simulink model "robosimulador"  (R2021b)
settings: Solver=VariableStepAuto  StartTime=0.0  StopTime=Time(length(Time))  MaxStep=1e-3  RelTol=1e-3
model workspace: external: MATLAB File /home/fabio/Desktop/Larc 2021/robosimulador_DataFile.m (data not in the file)
values from neighbouring files (symbols this model uses):
  j = length(Q)    [Cinematica_Comb.m]    (also in Cinematica_Heli_Coronal.m; Cinematica_Heli_Direta_Coronal.m; Cinematica_Heli_Sagital.m)
  Q = Qr    [Cinematica_Comb.m]
  X = zeros(1,14)    [Cinematica_Comb.m]    (also in Cinematica_Heli_Coronal.m = zeros(1,6); Cinematica_Heli_Direta_Coronal.m = zeros(1,6); Cinematica_Heli_Sagital.m = zeros(1,8))
  Y = zeros(1,14)    [Cinematica_Comb.m]    (also in Cinematica_Heli_Coronal.m = zeros(1,6); Cinematica_Heli_Direta_Coronal.m = zeros(1,6); Cinematica_Heli_Sagital.m = zeros(1,8))
  Z = zeros(1,14)    [Cinematica_Comb.m]    (also in Cinematica_Heli_Coronal.m = zeros(1,6); Cinematica_Heli_Direta_Coronal.m = zeros(1,6); Cinematica_Heli_Sagital.m = zeros(1,8))
undefined symbols (not defined in the file or in its folder): g, height_plane, plane_x, smiData, Time, Tmax, zzmp
libraries: nesl_utility x168, sm_lib x117, simulink x38, sharedutil x19, Contact_Forces_Lib x8
(part 1 of 6)
settings Model: Creator=fabio  LastModifiedBy=yurid
settings SolverCC: AlgebraicLoopSolver=TrustRegion
settings DebuggingCC: UnconnectedInputMsg=none  UnconnectedOutputMsg=none  SFMachineParentedDataDiag=warning
settings DiagnosticsConfigSet: SimMechanicsRigidlyBoundBlock=none

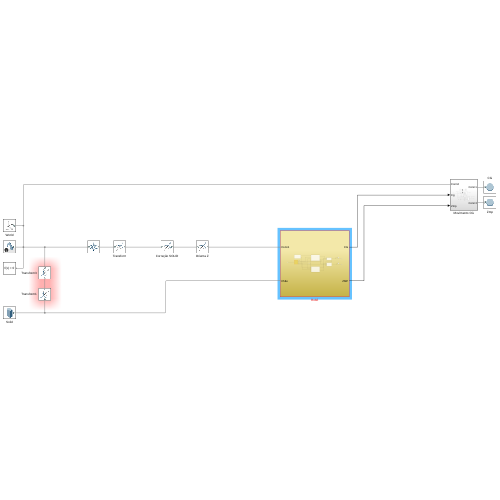
[thumbnail: Simulink's stored preview of the top-level diagram]
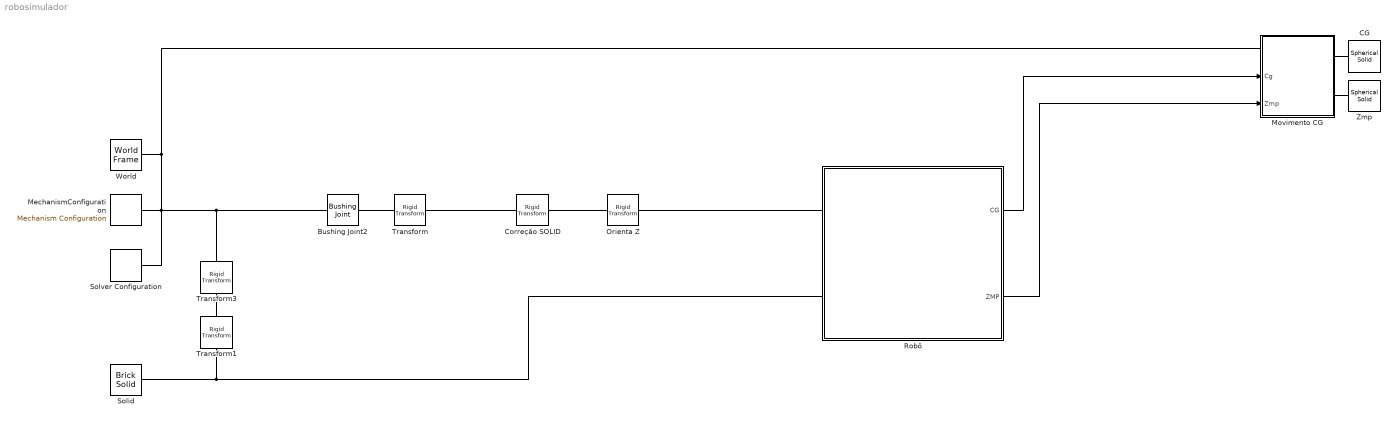
== system robosimulador ==
  Bushing Joint2 : sm_lib/Joints/Bushing Joint  JointMode=Normal  SenseConstraintForce=off  SenseConstraintForceX=off  SenseConstraintForceY=off  SenseConstraintForceZ=off  SenseConstraintTorque=off  SenseConstraintTorqueX=off  SenseConstraintTorqueY=off  SenseConstraintTorqueZ=off  SenseTotalForce=off  SenseTotalForceX=off  SenseTotalForceY=off  SenseTotalForceZ=off  SenseTotalTorque=off  SenseTotalTorqueX=off  SenseTotalTorqueY=off  SenseTotalTorqueZ=off  CompositeWrenchDir=FollowerOnBase  CompositeWrenchFrame=BaseFrame  PxEquilibriumPosition=0  PxEquilibriumPositionUnits=m  PxSpringStiffness=0  PxSpringStiffnessUnits=N/m  PxDampingCoefficient=0  PxDampingCoefficientUnits=N/(m/s)  PxTorqueActuationMode=NoTorque  PxMotionActuationMode=ComputedMotion  PxSensePosition=off  PxSenseVelocity=off  PxSenseAcceleration=off  PxSenseTorqueForce=off  PxSenseLowerLimitTorqueForce=off  PxSenseUpperLimitTorqueForce=off  PxLowerLimitSpecify=off  PxLowerLimitBound=-1  PxLowerLimitBoundUnits=m  PxLowerLimitStiffness=1e6  PxLowerLimitStiffnessUnits=N/m  PxLowerLimitDamping=1e3  PxLowerLimitDampingUnits=N/(m/s)  PxLowerLimitTransitionRegionWidth=1e-4  PxLowerLimitTransitionRegionWidthUnits=m  PxUpperLimitSpecify=off  PxUpperLimitBound=1  PxUpperLimitBoundUnits=m  PxUpperLimitStiffness=1e6  PxUpperLimitStiffnessUnits=N/m  PxUpperLimitDamping=1e3  PxUpperLimitDampingUnits=N/(m/s)  PxUpperLimitTransitionRegionWidth=1e-4  PxUpperLimitTransitionRegionWidthUnits=m  PxPositionTargetSpecify=off  PxPositionTargetPriority=High  PxPositionTargetValue=0  PxPositionTargetValueUnits=m  PxVelocityTargetSpecify=off  PxVelocityTargetPriority=High  PxVelocityTargetValue=0  PxVelocityTargetValueUnits=m/s  PyEquilibriumPosition=0  PyEquilibriumPositionUnits=m  PySpringStiffness=0  PySpringStiffnessUnits=N/m  PyDampingCoefficient=0  PyDampingCoefficientUnits=N/(m/s)  PyTorqueActuationMode=NoTorque  PyMotionActuationMode=ComputedMotion  PySensePosition=off  PySenseVelocity=off  PySenseAcceleration=off  PySenseTorqueForce=off  PySenseLowerLimitTorqueForce=off  PySenseUpperLimitTorqueForce=off  PyLowerLimitSpecify=off  PyLowerLimitBound=-1  PyLowerLimitBoundUnits=m  PyLowerLimitStiffness=1e6  PyLowerLimitStiffnessUnits=N/m  PyLowerLimitDamping=1e3  PyLowerLimitDampingUnits=N/(m/s)  PyLowerLimitTransitionRegionWidth=1e-4  PyLowerLimitTransitionRegionWidthUnits=m  PyUpperLimitSpecify=off  PyUpperLimitBound=1  PyUpperLimitBoundUnits=m  PyUpperLimitStiffness=1e6  PyUpperLimitStiffnessUnits=N/m  PyUpperLimitDamping=1e3  PyUpperLimitDampingUnits=N/(m/s)  PyUpperLimitTransitionRegionWidth=1e-4  PyUpperLimitTransitionRegionWidthUnits=m  PyPositionTargetSpecify=off  PyPositionTargetPriority=High  PyPositionTargetValue=0  PyPositionTargetValueUnits=m  PyVelocityTargetSpecify=off  PyVelocityTargetPriority=High  PyVelocityTargetValue=0  PyVelocityTargetValueUnits=m/s  PzEquilibriumPosition=0  PzEquilibriumPositionUnits=m  PzSpringStiffness=0  PzSpringStiffnessUnits=N/m  PzDampingCoefficient=0  PzDampingCoefficientUnits=N/(m/s)  PzTorqueActuationMode=NoTorque  PzMotionActuationMode=ComputedMotion  PzSensePosition=off  PzSenseVelocity=off  PzSenseAcceleration=off  PzSenseTorqueForce=off  PzSenseLowerLimitTorqueForce=off  PzSenseUpperLimitTorqueForce=off  PzLowerLimitSpecify=off  PzLowerLimitBound=-1  PzLowerLimitBoundUnits=m  PzLowerLimitStiffness=1e6  PzLowerLimitStiffnessUnits=N/m  PzLowerLimitDamping=1e3  PzLowerLimitDampingUnits=N/(m/s)  PzLowerLimitTransitionRegionWidth=1e-4  PzLowerLimitTransitionRegionWidthUnits=m  PzUpperLimitSpecify=off  PzUpperLimitBound=1  PzUpperLimitBoundUnits=m  PzUpperLimitStiffness=1e6  PzUpperLimitStiffnessUnits=N/m  PzUpperLimitDamping=1e3  PzUpperLimitDampingUnits=N/(m/s)  PzUpperLimitTransitionRegionWidth=1e-4  PzUpperLimitTransitionRegionWidthUnits=m  PzPositionTargetSpecify=off  PzPositionTargetPriority=High  PzPositionTargetValue=1  PzPositionTargetValueUnits=m  PzVelocityTargetSpecify=off  PzVelocityTargetPriority=High  PzVelocityTargetValue=0  PzVelocityTargetValueUnits=m/s  RxEquilibriumPosition=0  RxEquilibriumPositionUnits=deg  RxSpringStiffness=0  RxSpringStiffnessUnits=N*m/deg  RxDampingCoefficient=0  RxDampingCoefficientUnits=N*m/(deg/s)  RxTorqueActuationMode=NoTorque  RxMotionActuationMode=ComputedMotion  RxSensePosition=off  RxSenseVelocity=off  RxSenseAcceleration=off  RxSenseTorqueForce=off  RxSenseLowerLimitTorqueForce=off  RxSenseUpperLimitTorqueForce=off  RxLowerLimitSpecify=off  RxLowerLimitBound=-90  RxLowerLimitBoundUnits=deg  RxLowerLimitStiffness=1e4  RxLowerLimitStiffnessUnits=N*m/deg  RxLowerLimitDamping=10  RxLowerLimitDampingUnits=N*m/(deg/s)  RxLowerLimitTransitionRegionWidth=0.1  RxLowerLimitTransitionRegionWidthUnits=deg  RxUpperLimitSpecify=off  RxUpperLimitBound=90  RxUpperLimitBoundUnits=deg  RxUpperLimitStiffness=1e4  RxUpperLimitStiffnessUnits=N*m/deg  RxUpperLimitDamping=10  RxUpperLimitDampingUnits=N*m/(deg/s)  RxUpperLimitTransitionRegionWidth=0.1  RxUpperLimitTransitionRegionWidthUnits=deg  RxPositionTargetSpecify=off  RxPositionTargetPriority=High  RxPositionTargetValue=0  RxPositionTargetValueUnits=deg  RxVelocityTargetSpecify=off  RxVelocityTargetPriority=High  RxVelocityTargetValue=0  RxVelocityTargetValueUnits=deg/s  RyEquilibriumPosition=0  RyEquilibriumPositionUnits=deg  RySpringStiffness=0  RySpringStiffnessUnits=N*m/deg  RyDampingCoefficient=0  RyDampingCoefficientUnits=N*m/(deg/s)  RyTorqueActuationMode=NoTorque  RyMotionActuationMode=ComputedMotion  RySensePosition=off  RySenseVelocity=off  RySenseAcceleration=off  RySenseTorqueForce=off  RySenseLowerLimitTorqueForce=off  RySenseUpperLimitTorqueForce=off  RyLowerLimitSpecify=off  RyLowerLimitBound=-90  RyLowerLimitBoundUnits=deg  RyLowerLimitStiffness=1e4  RyLowerLimitStiffnessUnits=N*m/deg  RyLowerLimitDamping=10  RyLowerLimitDampingUnits=N*m/(deg/s)  RyLowerLimitTransitionRegionWidth=0.1  RyLowerLimitTransitionRegionWidthUnits=deg  RyUpperLimitSpecify=off  RyUpperLimitBound=90  RyUpperLimitBoundUnits=deg  RyUpperLimitStiffness=1e4  RyUpperLimitStiffnessUnits=N*m/deg  RyUpperLimitDamping=10  RyUpperLimitDampingUnits=N*m/(deg/s)  RyUpperLimitTransitionRegionWidth=0.1  RyUpperLimitTransitionRegionWidthUnits=deg  RyPositionTargetSpecify=off  RyPositionTargetPriority=High  RyPositionTargetValue=0  RyPositionTargetValueUnits=deg  RyVelocityTargetSpecify=off  RyVelocityTargetPriority=High  RyVelocityTargetValue=0  RyVelocityTargetValueUnits=deg/s  RzEquilibriumPosition=0  RzEquilibriumPositionUnits=deg  RzSpringStiffness=0  RzSpringStiffnessUnits=N*m/deg  RzDampingCoefficient=0  RzDampingCoefficientUnits=N*m/(deg/s)  RzTorqueActuationMode=NoTorque  RzMotionActuationMode=ComputedMotion  RzSensePosition=off  RzSenseVelocity=off  RzSenseAcceleration=off  RzSenseTorqueForce=off  RzSenseLowerLimitTorqueForce=off  RzSenseUpperLimitTorqueForce=off  RzLowerLimitSpecify=off  RzLowerLimitBound=-90  RzLowerLimitBoundUnits=deg  RzLowerLimitStiffness=1e4  RzLowerLimitStiffnessUnits=N*m/deg  RzLowerLimitDamping=10  RzLowerLimitDampingUnits=N*m/(deg/s)  RzLowerLimitTransitionRegionWidth=0.1  RzLowerLimitTransitionRegionWidthUnits=deg  RzUpperLimitSpecify=off  RzUpperLimitBound=90  RzUpperLimitBoundUnits=deg  RzUpperLimitStiffness=1e4  RzUpperLimitStiffnessUnits=N*m/deg  RzUpperLimitDamping=10  RzUpperLimitDampingUnits=N*m/(deg/s)  RzUpperLimitTransitionRegionWidth=0.1  RzUpperLimitTransitionRegionWidthUnits=deg  RzPositionTargetSpecify=off  RzPositionTargetPriority=High  RzPositionTargetValue=0  RzPositionTargetValueUnits=deg  RzVelocityTargetSpecify=off  RzVelocityTargetPriority=High  RzVelocityTargetValue=0  RzVelocityTargetValueUnits=deg/s
  CG : sm_lib/Body Elements/Spherical Solid  GraphicAmbientColor=[0.15 0.15 0.15 1.0]  BasedOnType=Density  CenterOfMass=[0 0 0]  CenterOfMassUnits=m  GraphicDiffuseColor=[0.2 1.0 0.0]  Density=1000  DensityUnits=kg/m^3  DoExposeReferenceFrame=on  GraphicEmissiveColor=[0.0 0.0 0.0 1.0]  ExportEntireGeometry=off  SerializedExposedGeometries=<ExposedGeometries/>  SerializedFrames=<Frames/>  MarkerShape=Sphere  MarkerSize=10  GraphicType=FromGeometry  InertiaType=CalculateFromGeometry  Mass=1  MassUnits=kg  MomentsOfInertia=[1 1 1]  MomentsOfInertiaUnits=kg*m^2  GraphicOpacity=1.0  ProductsOfInertia=[0 0 0]  ProductsOfInertiaUnits=kg*m^2  GraphicShininess=75  GraphicSpecularColor=[0.5 0.5 0.5 1.0]  SphereRadius=0.01  SphereRadiusUnits=m  GraphicVisPropType=SimpleVisualProperties
  Correção SOLID : sm_lib/Frames and Transforms/Rigid Transform  TranslationMethod=None  TranslationStandardOffset=0  TranslationLengthUnit=mm  TranslationStandardAxis=+Z  TranslationCartesianOffset=0  TranslationROffset=0  TranslationROffsetUnits=m  TranslationZOffset=0  TranslationZOffsetUnits=m  TranslationThetaOffset=0  TranslationThetaOffsetUnits=deg  RotationMethod=StandardAxis  RotationAngleUnits=deg  RotationStandardAxis=-Z  RotationAngle=13.6  RotationArbitraryAxis=0  FollAlignAxisA=+X  BaseAlignAxisA=+Y  FollAlignAxisB=+Y  BaseAlignAxisB=+Z  RotationSequenceAxes=FollowerAxes  RotationSequence=XYX  RotationSequenceAngles=[0 0 0]  RotationSequenceAnglesUnits=deg  RotationMatrix=[1 0 0; 0 1 0; 0 0 1]
  MechanismConfiguration : sm_lib/Utilities/Mechanism Configuration  UniformGravity=Constant  GravityVector=[0 0 -9.80665]  GravityUnits=m/s^2  LinearizationDelta=0.001  JointModeTransitionNonlinearIterations=2
  Movimento CG : Subsystem
      settings: PortSchema="{\"entries\":[{\"content\":{\"sides\":[{\"content\":{\"connectorIds\":[\"LConn1\",\"In1\",\"In2\"]},\"type\":\"ConnectorPlacement.EquallySpacedRectSide\",\"uuid\":\"e9e729ac-da44-45ac-96b7-74b9933617c8\"},{\"content\":{\"connectorIds\":[\"RConn1\",\"RConn2\"],\"side\":\"RIGHT\"},\"type\":\"ConnectorPlacement.EquallySpacedRectSide\",\"uuid\":\"b7965d14-34ef-45b5-990a-29849adbef07\"},{\"content\":{\"connectorIds\":[],\"side\":\"TOP\"},\"type\":\"ConnectorPlacement.EquallySpacedRectSide\",\"uuid\":\"174ef9aa-3bee-4810-8e13-2d3bbeb9af5d\"}]},\"type\":\"ConnectorPlacement.EquallySpacedConnector\",\"uuid\":\"22440da4-e6bb-4652-99bb-446a9d9c0133\"}],\"packageUris\":[\"http://schema.mathworks.com/mf0/Connector/R2020b\"],\"version\":\"1.0\"}"
  Orienta Z : sm_lib/Frames and Transforms/Rigid Transform  TranslationMethod=None  TranslationStandardOffset=0  TranslationLengthUnit=mm  TranslationStandardAxis=+Z  TranslationCartesianOffset=0  TranslationROffset=0  TranslationROffsetUnits=m  TranslationZOffset=0  TranslationZOffsetUnits=m  TranslationThetaOffset=0  TranslationThetaOffsetUnits=deg  RotationMethod=StandardAxis  RotationAngleUnits=deg  RotationStandardAxis=+Z  RotationAngle=90  RotationArbitraryAxis=0  FollAlignAxisA=+X  BaseAlignAxisA=+Y  FollAlignAxisB=+Y  BaseAlignAxisB=+Z  RotationSequenceAxes=FollowerAxes  RotationSequence=XYX  RotationSequenceAngles=[0 0 0]  RotationSequenceAnglesUnits=deg  RotationMatrix=[1 0 0; 0 1 0; 0 0 1]
  Robô : Subsystem
  Solid : sm_lib/Body Elements/Brick Solid  GraphicAmbientColor=[0.15 0.15 0.15 1.0]  BasedOnType=Density  BrickDimensions=chao  BrickDimensionUnits=m  CenterOfMass=[0 0 0]  CenterOfMassUnits=m  GraphicDiffuseColor=[0.5 0.5 0.5]  Density=1000  DensityUnits=kg/m^3  DoExposeReferenceFrame=on  GraphicEmissiveColor=[0.0 0.0 0.0 1.0]  ExportEntireGeometry=off  SerializedFrames=<Frames/>  MarkerShape=Sphere  MarkerSize=10  GraphicType=FromGeometry  InertiaType=CalculateFromGeometry  Mass=1  MassUnits=kg  MomentsOfInertia=[1 1 1]  MomentsOfInertiaUnits=kg*m^2  GraphicOpacity=1.0  ProductsOfInertia=[0 0 0]  ProductsOfInertiaUnits=kg*m^2  GraphicShininess=75  GraphicSpecularColor=[0.5 0.5 0.5 1.0]  GraphicVisPropType=SimpleVisualProperties
  Solver Configuration : nesl_utility/Solver Configuration  PhysicalDomain=network_engine_domain  SubClassName=solver  LeftPortType=input  RightPortType=generic  Tones=[]  Harmonics=[]  SimulateNoise=off  Profile=off  UseLocalSampling=off  EnableSwitchedLinearOptims=on  FrequencyDomain=off  UseCCode=off  RelTol=0.001  AbsTol=1e-06  MinStep=1e-09  ToWorkspace=off  RevertToSquareIcSolve=off  NumHomotopyIterations=100  PhasorMode=off  PhasorModeNumHarmonics=1  DoDC=off  ResidualTolerance=1e-09  UseLocalSolver=off  LocalSolverChoice=NE_BACKWARD_EULER_ADVANCER  LocalSolverSampleTime=0.001  DoFixedCost=off  MaxNonlinIter=3  MaxModeIter=2  ComputeImpulses=off  ImpulseIterations=2  LinearAlgebra=auto  EquationFormulation=NE_TIME_EF  DelaysMemoryBudget=1024  AutomaticFiltering=on  FilteringTimeConstant=0.001  PartitionStorageMethod=AS_NEEDED  PartitionMemoryBudget=1024  PartitionMethod=ROBUST
      settings: SourceProductBaseCode=PW,SS
  Transform : sm_lib/Frames and Transforms/Rigid Transform  TranslationMethod=Cartesian  TranslationStandardOffset=0  TranslationLengthUnit=mm  TranslationStandardAxis=+Z  TranslationCartesianOffset=smiData.RigidTransform(37).translation  TranslationROffset=0  TranslationROffsetUnits=m  TranslationZOffset=0  TranslationZOffsetUnits=m  TranslationThetaOffset=0  TranslationThetaOffsetUnits=deg  RotationMethod=ArbitraryAxis  RotationAngleUnits=rad  RotationStandardAxis=+Z  RotationAngle=smiData.RigidTransform(37).angle  RotationArbitraryAxis=smiData.RigidTransform(37).axis  FollAlignAxisA=+X  BaseAlignAxisA=+Y  FollAlignAxisB=+Y  BaseAlignAxisB=+Z  RotationSequenceAxes=FollowerAxes  RotationSequence=XYX  RotationSequenceAngles=[0 0 0]  RotationSequenceAnglesUnits=deg  RotationMatrix=[1 0 0; 0 1 0; 0 0 1]
  Transform1 : sm_lib/Frames and Transforms/Rigid Transform  TranslationMethod=StandardAxis  TranslationStandardOffset=plane_x/2-0.2  TranslationLengthUnit=m  TranslationStandardAxis=+X  TranslationCartesianOffset=0.2  TranslationROffset=0  TranslationROffsetUnits=m  TranslationZOffset=0  TranslationZOffsetUnits=m  TranslationThetaOffset=0  TranslationThetaOffsetUnits=deg  RotationMethod=None  RotationAngleUnits=deg  RotationStandardAxis=+X  RotationAngle=90  RotationArbitraryAxis=smiData.RigidTransform(23).axis  FollAlignAxisA=+X  BaseAlignAxisA=+Y  FollAlignAxisB=+Y  BaseAlignAxisB=+Z  RotationSequenceAxes=FollowerAxes  RotationSequence=XYX  RotationSequenceAngles=[0 0 0]  RotationSequenceAnglesUnits=deg  RotationMatrix=[1 0 0; 0 1 0; 0 0 1]
  Transform3 : sm_lib/Frames and Transforms/Rigid Transform  TranslationMethod=StandardAxis  TranslationStandardOffset=dz  TranslationLengthUnit=m  TranslationStandardAxis=+Z  TranslationCartesianOffset=0.2  TranslationROffset=0  TranslationROffsetUnits=m  TranslationZOffset=0  TranslationZOffsetUnits=m  TranslationThetaOffset=0  TranslationThetaOffsetUnits=deg  RotationMethod=None  RotationAngleUnits=deg  RotationStandardAxis=+X  RotationAngle=90  RotationArbitraryAxis=smiData.RigidTransform(23).axis  FollAlignAxisA=+X  BaseAlignAxisA=+Y  FollAlignAxisB=+Y  BaseAlignAxisB=+Z  RotationSequenceAxes=FollowerAxes  RotationSequence=XYX  RotationSequenceAngles=[0 0 0]  RotationSequenceAnglesUnits=deg  RotationMatrix=[1 0 0; 0 1 0; 0 0 1]
  World : sm_lib/Frames and Transforms/World Frame
  Zmp : sm_lib/Body Elements/Spherical Solid  GraphicAmbientColor=[0.15 0.15 0.15 1.0]  BasedOnType=Density  CenterOfMass=[0 0 0]  CenterOfMassUnits=m  GraphicDiffuseColor=[1.0 0.0 0.0]  Density=1000  DensityUnits=kg/m^3  DoExposeReferenceFrame=on  GraphicEmissiveColor=[0.0 0.0 0.0 1.0]  ExportEntireGeometry=off  SerializedExposedGeometries=<ExposedGeometries/>  SerializedFrames=<Frames/>  MarkerShape=Sphere  MarkerSize=10  GraphicType=FromGeometry  InertiaType=CalculateFromGeometry  Mass=1  MassUnits=kg  MomentsOfInertia=[1 1 1]  MomentsOfInertiaUnits=kg*m^2  GraphicOpacity=1.0  ProductsOfInertia=[0 0 0]  ProductsOfInertiaUnits=kg*m^2  GraphicShininess=75  GraphicSpecularColor=[0.5 0.5 0.5 1.0]  SphereRadius=0.01  SphereRadiusUnits=m  GraphicVisPropType=SimpleVisualProperties
  wires:
  Robô/2(ZMP) -> Movimento CG/2(Zmp)
  Robô/1(CG) -> Movimento CG/1(Cg)
  connections:
  MechanismConfiguration/RConn1 -- Solver Configuration/RConn1 -- Movimento CG/LConn1 -- World/RConn1 -- Bushing Joint2/LConn1 -- Transform3/LConn1
  Robô/LConn1 -- Orienta Z/RConn1
  Correção SOLID/LConn1 -- Transform/RConn1
  Orienta Z/LConn1 -- Correção SOLID/RConn1
  Transform3/RConn1 -- Transform1/LConn1
  Transform1/RConn1 -- Robô/LConn2 -- Solid/RConn1
  Bushing Joint2/RConn1 -- Transform/LConn1
  CG/RConn1 -- Movimento CG/RConn1
  Zmp/RConn1 -- Movimento CG/RConn2

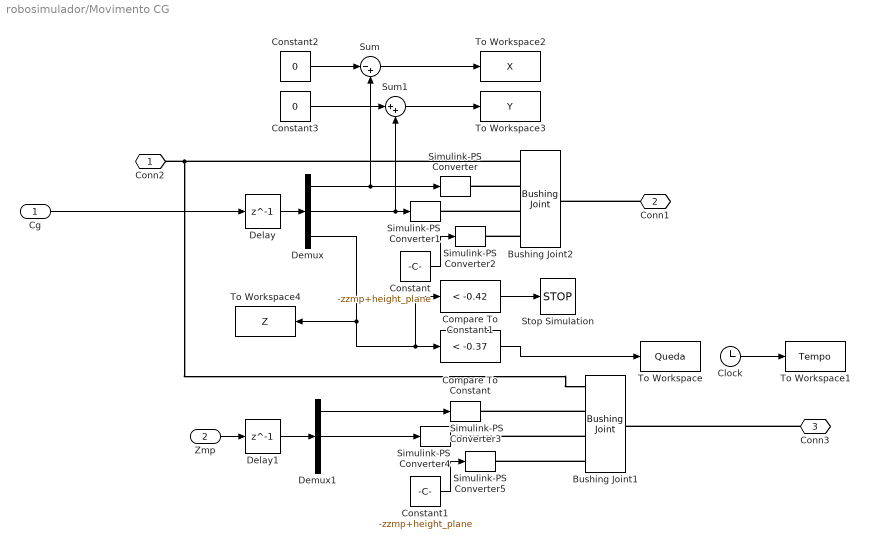
== system robosimulador/Movimento CG ==
  Cg : Inport
  Zmp : Inport  Port=2
  Bushing Joint1 : sm_lib/Joints/Bushing Joint  JointMode=Normal  SenseConstraintForce=off  SenseConstraintForceX=off  SenseConstraintForceY=off  SenseConstraintForceZ=off  SenseConstraintTorque=off  SenseConstraintTorqueX=off  SenseConstraintTorqueY=off  SenseConstraintTorqueZ=off  SenseTotalForce=off  SenseTotalForceX=off  SenseTotalForceY=off  SenseTotalForceZ=off  SenseTotalTorque=off  SenseTotalTorqueX=off  SenseTotalTorqueY=off  SenseTotalTorqueZ=off  CompositeWrenchDir=FollowerOnBase  CompositeWrenchFrame=BaseFrame  PxEquilibriumPosition=0  PxEquilibriumPositionUnits=m  PxSpringStiffness=0  PxSpringStiffnessUnits=N/m  PxDampingCoefficient=0  PxDampingCoefficientUnits=N/(m/s)  PxTorqueActuationMode=ComputedTorque  PxMotionActuationMode=InputMotion  PxSensePosition=off  PxSenseVelocity=off  PxSenseAcceleration=off  PxSenseTorqueForce=off  PxSenseLowerLimitTorqueForce=off  PxSenseUpperLimitTorqueForce=off  PxLowerLimitSpecify=off  PxLowerLimitBound=-1  PxLowerLimitBoundUnits=m  PxLowerLimitStiffness=1e6  PxLowerLimitStiffnessUnits=N/m  PxLowerLimitDamping=1e3  PxLowerLimitDampingUnits=N/(m/s)  PxLowerLimitTransitionRegionWidth=1e-4  PxLowerLimitTransitionRegionWidthUnits=m  PxUpperLimitSpecify=off  PxUpperLimitBound=1  PxUpperLimitBoundUnits=m  PxUpperLimitStiffness=1e6  PxUpperLimitStiffnessUnits=N/m  PxUpperLimitDamping=1e3  PxUpperLimitDampingUnits=N/(m/s)  PxUpperLimitTransitionRegionWidth=1e-4  PxUpperLimitTransitionRegionWidthUnits=m  PxPositionTargetSpecify=off  PxPositionTargetPriority=High  PxPositionTargetValue=0  PxPositionTargetValueUnits=m  PxVelocityTargetSpecify=off  PxVelocityTargetPriority=High  PxVelocityTargetValue=0  PxVelocityTargetValueUnits=m/s  PyEquilibriumPosition=0  PyEquilibriumPositionUnits=m  PySpringStiffness=0  PySpringStiffnessUnits=N/m  PyDampingCoefficient=0  PyDampingCoefficientUnits=N/(m/s)  PyTorqueActuationMode=ComputedTorque  PyMotionActuationMode=InputMotion  PySensePosition=off  PySenseVelocity=off  PySenseAcceleration=off  PySenseTorqueForce=off  PySenseLowerLimitTorqueForce=off  PySenseUpperLimitTorqueForce=off  PyLowerLimitSpecify=off  PyLowerLimitBound=-1  PyLowerLimitBoundUnits=m  PyLowerLimitStiffness=1e6  PyLowerLimitStiffnessUnits=N/m  PyLowerLimitDamping=1e3  PyLowerLimitDampingUnits=N/(m/s)  PyLowerLimitTransitionRegionWidth=1e-4  PyLowerLimitTransitionRegionWidthUnits=m  PyUpperLimitSpecify=off  PyUpperLimitBound=1  PyUpperLimitBoundUnits=m  PyUpperLimitStiffness=1e6  PyUpperLimitStiffnessUnits=N/m  PyUpperLimitDamping=1e3  PyUpperLimitDampingUnits=N/(m/s)  PyUpperLimitTransitionRegionWidth=1e-4  PyUpperLimitTransitionRegionWidthUnits=m  PyPositionTargetSpecify=off  PyPositionTargetPriority=High  PyPositionTargetValue=0  PyPositionTargetValueUnits=m  PyVelocityTargetSpecify=off  PyVelocityTargetPriority=High  PyVelocityTargetValue=0  PyVelocityTargetValueUnits=m/s  PzEquilibriumPosition=0  PzEquilibriumPositionUnits=m  PzSpringStiffness=0  PzSpringStiffnessUnits=N/m  PzDampingCoefficient=0  PzDampingCoefficientUnits=N/(m/s)  PzTorqueActuationMode=ComputedTorque  PzMotionActuationMode=InputMotion  PzSensePosition=off  PzSenseVelocity=off  PzSenseAcceleration=off  PzSenseTorqueForce=off  PzSenseLowerLimitTorqueForce=off  PzSenseUpperLimitTorqueForce=off  PzLowerLimitSpecify=off  PzLowerLimitBound=-1  PzLowerLimitBoundUnits=m  PzLowerLimitStiffness=1e6  PzLowerLimitStiffnessUnits=N/m  PzLowerLimitDamping=1e3  PzLowerLimitDampingUnits=N/(m/s)  PzLowerLimitTransitionRegionWidth=1e-4  PzLowerLimitTransitionRegionWidthUnits=m  PzUpperLimitSpecify=off  PzUpperLimitBound=1  PzUpperLimitBoundUnits=m  PzUpperLimitStiffness=1e6  PzUpperLimitStiffnessUnits=N/m  PzUpperLimitDamping=1e3  PzUpperLimitDampingUnits=N/(m/s)  PzUpperLimitTransitionRegionWidth=1e-4  PzUpperLimitTransitionRegionWidthUnits=m  PzPositionTargetSpecify=off  PzPositionTargetPriority=High  PzPositionTargetValue=1  PzPositionTargetValueUnits=m  PzVelocityTargetSpecify=off  PzVelocityTargetPriority=High  PzVelocityTargetValue=0  PzVelocityTargetValueUnits=m/s  RxEquilibriumPosition=0  RxEquilibriumPositionUnits=deg  RxSpringStiffness=0  RxSpringStiffnessUnits=N*m/deg  RxDampingCoefficient=0  RxDampingCoefficientUnits=N*m/(deg/s)  RxTorqueActuationMode=NoTorque  RxMotionActuationMode=ComputedMotion  RxSensePosition=off  RxSenseVelocity=off  RxSenseAcceleration=off  RxSenseTorqueForce=off  RxSenseLowerLimitTorqueForce=off  RxSenseUpperLimitTorqueForce=off  RxLowerLimitSpecify=off  RxLowerLimitBound=-90  RxLowerLimitBoundUnits=deg  RxLowerLimitStiffness=1e4  RxLowerLimitStiffnessUnits=N*m/deg  RxLowerLimitDamping=10  RxLowerLimitDampingUnits=N*m/(deg/s)  RxLowerLimitTransitionRegionWidth=0.1  RxLowerLimitTransitionRegionWidthUnits=deg  RxUpperLimitSpecify=off  RxUpperLimitBound=90  RxUpperLimitBoundUnits=deg  RxUpperLimitStiffness=1e4  RxUpperLimitStiffnessUnits=N*m/deg  RxUpperLimitDamping=10  RxUpperLimitDampingUnits=N*m/(deg/s)  RxUpperLimitTransitionRegionWidth=0.1  RxUpperLimitTransitionRegionWidthUnits=deg  RxPositionTargetSpecify=off  RxPositionTargetPriority=High  RxPositionTargetValue=0  RxPositionTargetValueUnits=deg  RxVelocityTargetSpecify=off  RxVelocityTargetPriority=High  RxVelocityTargetValue=0  RxVelocityTargetValueUnits=deg/s  RyEquilibriumPosition=0  RyEquilibriumPositionUnits=deg  RySpringStiffness=0  RySpringStiffnessUnits=N*m/deg  RyDampingCoefficient=0  RyDampingCoefficientUnits=N*m/(deg/s)  RyTorqueActuationMode=NoTorque  RyMotionActuationMode=ComputedMotion  RySensePosition=off  RySenseVelocity=off  RySenseAcceleration=off  RySenseTorqueForce=off  RySenseLowerLimitTorqueForce=off  RySenseUpperLimitTorqueForce=off  RyLowerLimitSpecify=off  RyLowerLimitBound=-90  RyLowerLimitBoundUnits=deg  RyLowerLimitStiffness=1e4  RyLowerLimitStiffnessUnits=N*m/deg  RyLowerLimitDamping=10  RyLowerLimitDampingUnits=N*m/(deg/s)  RyLowerLimitTransitionRegionWidth=0.1  RyLowerLimitTransitionRegionWidthUnits=deg  RyUpperLimitSpecify=off  RyUpperLimitBound=90  RyUpperLimitBoundUnits=deg  RyUpperLimitStiffness=1e4  RyUpperLimitStiffnessUnits=N*m/deg  RyUpperLimitDamping=10  RyUpperLimitDampingUnits=N*m/(deg/s)  RyUpperLimitTransitionRegionWidth=0.1  RyUpperLimitTransitionRegionWidthUnits=deg  RyPositionTargetSpecify=off  RyPositionTargetPriority=High  RyPositionTargetValue=0  RyPositionTargetValueUnits=deg  RyVelocityTargetSpecify=off  RyVelocityTargetPriority=High  RyVelocityTargetValue=0  RyVelocityTargetValueUnits=deg/s  RzEquilibriumPosition=0  RzEquilibriumPositionUnits=deg  RzSpringStiffness=0  RzSpringStiffnessUnits=N*m/deg  RzDampingCoefficient=0  RzDampingCoefficientUnits=N*m/(deg/s)  RzTorqueActuationMode=NoTorque  RzMotionActuationMode=ComputedMotion  RzSensePosition=off  RzSenseVelocity=off  RzSenseAcceleration=off  RzSenseTorqueForce=off  RzSenseLowerLimitTorqueForce=off  RzSenseUpperLimitTorqueForce=off  RzLowerLimitSpecify=off  RzLowerLimitBound=-90  RzLowerLimitBoundUnits=deg  RzLowerLimitStiffness=1e4  RzLowerLimitStiffnessUnits=N*m/deg  RzLowerLimitDamping=10  RzLowerLimitDampingUnits=N*m/(deg/s)  RzLowerLimitTransitionRegionWidth=0.1  RzLowerLimitTransitionRegionWidthUnits=deg  RzUpperLimitSpecify=off  RzUpperLimitBound=90  RzUpperLimitBoundUnits=deg  RzUpperLimitStiffness=1e4  RzUpperLimitStiffnessUnits=N*m/deg  RzUpperLimitDamping=10  RzUpperLimitDampingUnits=N*m/(deg/s)  RzUpperLimitTransitionRegionWidth=0.1  RzUpperLimitTransitionRegionWidthUnits=deg  RzPositionTargetSpecify=off  RzPositionTargetPriority=High  RzPositionTargetValue=0  RzPositionTargetValueUnits=deg  RzVelocityTargetSpecify=off  RzVelocityTargetPriority=High  RzVelocityTargetValue=0  RzVelocityTargetValueUnits=deg/s
  Bushing Joint2 : sm_lib/Joints/Bushing Joint  JointMode=Normal  SenseConstraintForce=off  SenseConstraintForceX=off  SenseConstraintForceY=off  SenseConstraintForceZ=off  SenseConstraintTorque=off  SenseConstraintTorqueX=off  SenseConstraintTorqueY=off  SenseConstraintTorqueZ=off  SenseTotalForce=off  SenseTotalForceX=off  SenseTotalForceY=off  SenseTotalForceZ=off  SenseTotalTorque=off  SenseTotalTorqueX=off  SenseTotalTorqueY=off  SenseTotalTorqueZ=off  CompositeWrenchDir=FollowerOnBase  CompositeWrenchFrame=BaseFrame  PxEquilibriumPosition=0  PxEquilibriumPositionUnits=m  PxSpringStiffness=0  PxSpringStiffnessUnits=N/m  PxDampingCoefficient=0  PxDampingCoefficientUnits=N/(m/s)  PxTorqueActuationMode=ComputedTorque  PxMotionActuationMode=InputMotion  PxSensePosition=off  PxSenseVelocity=off  PxSenseAcceleration=off  PxSenseTorqueForce=off  PxSenseLowerLimitTorqueForce=off  PxSenseUpperLimitTorqueForce=off  PxLowerLimitSpecify=off  PxLowerLimitBound=-1  PxLowerLimitBoundUnits=m  PxLowerLimitStiffness=1e6  PxLowerLimitStiffnessUnits=N/m  PxLowerLimitDamping=1e3  PxLowerLimitDampingUnits=N/(m/s)  PxLowerLimitTransitionRegionWidth=1e-4  PxLowerLimitTransitionRegionWidthUnits=m  PxUpperLimitSpecify=off  PxUpperLimitBound=1  PxUpperLimitBoundUnits=m  PxUpperLimitStiffness=1e6  PxUpperLimitStiffnessUnits=N/m  PxUpperLimitDamping=1e3  PxUpperLimitDampingUnits=N/(m/s)  PxUpperLimitTransitionRegionWidth=1e-4  PxUpperLimitTransitionRegionWidthUnits=m  PxPositionTargetSpecify=off  PxPositionTargetPriority=High  PxPositionTargetValue=0  PxPositionTargetValueUnits=m  PxVelocityTargetSpecify=off  PxVelocityTargetPriority=High  PxVelocityTargetValue=0  PxVelocityTargetValueUnits=m/s  PyEquilibriumPosition=0  PyEquilibriumPositionUnits=m  PySpringStiffness=0  PySpringStiffnessUnits=N/m  PyDampingCoefficient=0  PyDampingCoefficientUnits=N/(m/s)  PyTorqueActuationMode=ComputedTorque  PyMotionActuationMode=InputMotion  PySensePosition=off  PySenseVelocity=off  PySenseAcceleration=off  PySenseTorqueForce=off  PySenseLowerLimitTorqueForce=off  PySenseUpperLimitTorqueForce=off  PyLowerLimitSpecify=off  PyLowerLimitBound=-1  PyLowerLimitBoundUnits=m  PyLowerLimitStiffness=1e6  PyLowerLimitStiffnessUnits=N/m  PyLowerLimitDamping=1e3  PyLowerLimitDampingUnits=N/(m/s)  PyLowerLimitTransitionRegionWidth=1e-4  PyLowerLimitTransitionRegionWidthUnits=m  PyUpperLimitSpecify=off  PyUpperLimitBound=1  PyUpperLimitBoundUnits=m  PyUpperLimitStiffness=1e6  PyUpperLimitStiffnessUnits=N/m  PyUpperLimitDamping=1e3  PyUpperLimitDampingUnits=N/(m/s)  PyUpperLimitTransitionRegionWidth=1e-4  PyUpperLimitTransitionRegionWidthUnits=m  PyPositionTargetSpecify=off  PyPositionTargetPriority=High  PyPositionTargetValue=0  PyPositionTargetValueUnits=m  PyVelocityTargetSpecify=off  PyVelocityTargetPriority=High  PyVelocityTargetValue=0  PyVelocityTargetValueUnits=m/s  PzEquilibriumPosition=0  PzEquilibriumPositionUnits=m  PzSpringStiffness=0  PzSpringStiffnessUnits=N/m  PzDampingCoefficient=0  PzDampingCoefficientUnits=N/(m/s)  PzTorqueActuationMode=ComputedTorque  PzMotionActuationMode=InputMotion  PzSensePosition=off  PzSenseVelocity=off  PzSenseAcceleration=off  PzSenseTorqueForce=off  PzSenseLowerLimitTorqueForce=off  PzSenseUpperLimitTorqueForce=off  PzLowerLimitSpecify=off  PzLowerLimitBound=-1  PzLowerLimitBoundUnits=m  PzLowerLimitStiffness=1e6  PzLowerLimitStiffnessUnits=N/m  PzLowerLimitDamping=1e3  PzLowerLimitDampingUnits=N/(m/s)  PzLowerLimitTransitionRegionWidth=1e-4  PzLowerLimitTransitionRegionWidthUnits=m  PzUpperLimitSpecify=off  PzUpperLimitBound=1  PzUpperLimitBoundUnits=m  PzUpperLimitStiffness=1e6  PzUpperLimitStiffnessUnits=N/m  PzUpperLimitDamping=1e3  PzUpperLimitDampingUnits=N/(m/s)  PzUpperLimitTransitionRegionWidth=1e-4  PzUpperLimitTransitionRegionWidthUnits=m  PzPositionTargetSpecify=off  PzPositionTargetPriority=High  PzPositionTargetValue=1  PzPositionTargetValueUnits=m  PzVelocityTargetSpecify=off  PzVelocityTargetPriority=High  PzVelocityTargetValue=0  PzVelocityTargetValueUnits=m/s  RxEquilibriumPosition=0  RxEquilibriumPositionUnits=deg  RxSpringStiffness=0  RxSpringStiffnessUnits=N*m/deg  RxDampingCoefficient=0  RxDampingCoefficientUnits=N*m/(deg/s)  RxTorqueActuationMode=NoTorque  RxMotionActuationMode=ComputedMotion  RxSensePosition=off  RxSenseVelocity=off  RxSenseAcceleration=off  RxSenseTorqueForce=off  RxSenseLowerLimitTorqueForce=off  RxSenseUpperLimitTorqueForce=off  RxLowerLimitSpecify=off  RxLowerLimitBound=-90  RxLowerLimitBoundUnits=deg  RxLowerLimitStiffness=1e4  RxLowerLimitStiffnessUnits=N*m/deg  RxLowerLimitDamping=10  RxLowerLimitDampingUnits=N*m/(deg/s)  RxLowerLimitTransitionRegionWidth=0.1  RxLowerLimitTransitionRegionWidthUnits=deg  RxUpperLimitSpecify=off  RxUpperLimitBound=90  RxUpperLimitBoundUnits=deg  RxUpperLimitStiffness=1e4  RxUpperLimitStiffnessUnits=N*m/deg  RxUpperLimitDamping=10  RxUpperLimitDampingUnits=N*m/(deg/s)  RxUpperLimitTransitionRegionWidth=0.1  RxUpperLimitTransitionRegionWidthUnits=deg  RxPositionTargetSpecify=off  RxPositionTargetPriority=High  RxPositionTargetValue=0  RxPositionTargetValueUnits=deg  RxVelocityTargetSpecify=off  RxVelocityTargetPriority=High  RxVelocityTargetValue=0  RxVelocityTargetValueUnits=deg/s  RyEquilibriumPosition=0  RyEquilibriumPositionUnits=deg  RySpringStiffness=0  RySpringStiffnessUnits=N*m/deg  RyDampingCoefficient=0  RyDampingCoefficientUnits=N*m/(deg/s)  RyTorqueActuationMode=NoTorque  RyMotionActuationMode=ComputedMotion  RySensePosition=off  RySenseVelocity=off  RySenseAcceleration=off  RySenseTorqueForce=off  RySenseLowerLimitTorqueForce=off  RySenseUpperLimitTorqueForce=off  RyLowerLimitSpecify=off  RyLowerLimitBound=-90  RyLowerLimitBoundUnits=deg  RyLowerLimitStiffness=1e4  RyLowerLimitStiffnessUnits=N*m/deg  RyLowerLimitDamping=10  RyLowerLimitDampingUnits=N*m/(deg/s)  RyLowerLimitTransitionRegionWidth=0.1  RyLowerLimitTransitionRegionWidthUnits=deg  RyUpperLimitSpecify=off  RyUpperLimitBound=90  RyUpperLimitBoundUnits=deg  RyUpperLimitStiffness=1e4  RyUpperLimitStiffnessUnits=N*m/deg  RyUpperLimitDamping=10  RyUpperLimitDampingUnits=N*m/(deg/s)  RyUpperLimitTransitionRegionWidth=0.1  RyUpperLimitTransitionRegionWidthUnits=deg  RyPositionTargetSpecify=off  RyPositionTargetPriority=High  RyPositionTargetValue=0  RyPositionTargetValueUnits=deg  RyVelocityTargetSpecify=off  RyVelocityTargetPriority=High  RyVelocityTargetValue=0  RyVelocityTargetValueUnits=deg/s  RzEquilibriumPosition=0  RzEquilibriumPositionUnits=deg  RzSpringStiffness=0  RzSpringStiffnessUnits=N*m/deg  RzDampingCoefficient=0  RzDampingCoefficientUnits=N*m/(deg/s)  RzTorqueActuationMode=NoTorque  RzMotionActuationMode=ComputedMotion  RzSensePosition=off  RzSenseVelocity=off  RzSenseAcceleration=off  RzSenseTorqueForce=off  RzSenseLowerLimitTorqueForce=off  RzSenseUpperLimitTorqueForce=off  RzLowerLimitSpecify=off  RzLowerLimitBound=-90  RzLowerLimitBoundUnits=deg  RzLowerLimitStiffness=1e4  RzLowerLimitStiffnessUnits=N*m/deg  RzLowerLimitDamping=10  RzLowerLimitDampingUnits=N*m/(deg/s)  RzLowerLimitTransitionRegionWidth=0.1  RzLowerLimitTransitionRegionWidthUnits=deg  RzUpperLimitSpecify=off  RzUpperLimitBound=90  RzUpperLimitBoundUnits=deg  RzUpperLimitStiffness=1e4  RzUpperLimitStiffnessUnits=N*m/deg  RzUpperLimitDamping=10  RzUpperLimitDampingUnits=N*m/(deg/s)  RzUpperLimitTransitionRegionWidth=0.1  RzUpperLimitTransitionRegionWidthUnits=deg  RzPositionTargetSpecify=off  RzPositionTargetPriority=High  RzPositionTargetValue=0  RzPositionTargetValueUnits=deg  RzVelocityTargetSpecify=off  RzVelocityTargetPriority=High  RzVelocityTargetValue=0  RzVelocityTargetValueUnits=deg/s
  Clock : Clock
  Compare To Constant : simulink/Logic and Bit Operations/Compare To Constant  relop=<  const=-0.37  OutDataTypeStr=boolean
  Compare To Constant1 : simulink/Logic and Bit Operations/Compare To Constant  relop=<  const=-0.42  OutDataTypeStr=boolean
  Constant : Constant  Value=-zzmp+height_plane
  Constant1 : Constant  Value=-zzmp+height_plane
  Constant2 : Constant  Value=0
  Constant3 : Constant  Value=0
  Delay : Delay  DelayLength=1  InitialCondition=0
  Delay1 : Delay  DelayLength=1  InitialCondition=0
  Demux : Demux  Outputs=3
  Demux1 : Demux  Outputs=3
  Simulink-PS Converter : nesl_utility/Simulink-PS Converter  PhysicalDomain=network_engine_domain  SubClassName=ps_input  LeftPortType=input  RightPortType=output  PseudoPeriodic=off  Frequencies=[]  NoiseDistribution=none  NoiseParameters=[]  Unit=m  AffineConversion=off  FilteringAndDerivatives=filter  SimscapeFilterOrder=2  InputFilterTimeConstant=0.01  UdotUserProvided=2
      settings: SourceProductBaseCode=PW,SS
  Simulink-PS Converter{1..2,4..5} (4 alike) : nesl_utility/Simulink-PS Converter  PhysicalDomain=network_engine_domain  SubClassName=ps_input  LeftPortType=input  RightPortType=output  PseudoPeriodic=off  Frequencies=[]  NoiseDistribution=none  NoiseParameters=[]  Unit=m  AffineConversion=off  FilteringAndDerivatives=filter  SimscapeFilterOrder=2  InputFilterTimeConstant=0.01  UdotUserProvided=0
      settings: SourceProductBaseCode=PW,SS
  Simulink-PS Converter3 : nesl_utility/Simulink-PS Converter  PhysicalDomain=network_engine_domain  SubClassName=ps_input  LeftPortType=input  RightPortType=output  PseudoPeriodic=off  Frequencies=[]  NoiseDistribution=none  NoiseParameters=[]  Unit=m  AffineConversion=off  FilteringAndDerivatives=filter  SimscapeFilterOrder=2  InputFilterTimeConstant=0.01  UdotUserProvided=2
      settings: SourceProductBaseCode=PW,SS
  Stop Simulation : Stop
  Sum : Sum  Inputs=|-+
  Sum1 : Sum  Inputs=|++
  To Workspace : ToWorkspace  VariableName=Queda  SampleTime=-1
      settings: Save2DSignal=2-D array (concatenate along first dimension)
  To Workspace1 : ToWorkspace  VariableName=Tempo  SampleTime=-1
      settings: Save2DSignal=2-D array (concatenate along first dimension)
  To Workspace2 : ToWorkspace  VariableName=X  SampleTime=-1
      settings: Save2DSignal=2-D array (concatenate along first dimension)
  To Workspace3 : ToWorkspace  VariableName=Y  SampleTime=-1
      settings: Save2DSignal=2-D array (concatenate along first dimension)
  To Workspace4 : ToWorkspace  VariableName=Z  SampleTime=-1
      settings: Save2DSignal=2-D array (concatenate along first dimension)
  Conn2 : PMIOPort  Side=Left
  Conn1 : PMIOPort  Port=2  Side=Right
  Conn3 : PMIOPort  Port=3  Side=Right
  wires:
  Constant/1 -> Simulink-PS Converter2/1
  Compare To Constant/1 -> To Workspace/1
  Constant1/1 -> Simulink-PS Converter5/1
  Cg/1 -> Delay/1
  Delay/1 -> Demux/1
  Demux/2 -> Sum1/2, Simulink-PS Converter1/1
  Demux/1 -> Sum/2, Simulink-PS Converter/1
  Zmp/1 -> Delay1/1
  Delay1/1 -> Demux1/1
  Demux1/1 -> Simulink-PS Converter3/1
  Demux1/2 -> Simulink-PS Converter4/1
  Clock/1 -> To Workspace1/1
  Demux/3 -> To Workspace4/1, Compare To Constant1/1, Compare To Constant/1
  Sum/1 -> To Workspace2/1
  Constant2/1 -> Sum/1
  Sum1/1 -> To Workspace3/1
  Constant3/1 -> Sum1/1
  Compare To Constant1/1 -> Stop Simulation/1
  connections:
  Bushing Joint2/LConn3 -- Simulink-PS Converter1/RConn1
  Bushing Joint2/LConn4 -- Simulink-PS Converter2/RConn1
  Conn1/RConn1 -- Bushing Joint2/RConn1
  Bushing Joint2/LConn2 -- Simulink-PS Converter/RConn1
  Conn3/RConn1 -- Bushing Joint1/RConn1
  Bushing Joint1/LConn2 -- Simulink-PS Converter3/RConn1
  Bushing Joint1/LConn4 -- Simulink-PS Converter5/RConn1
  Bushing Joint1/LConn3 -- Simulink-PS Converter4/RConn1
  Bushing Joint2/LConn1 -- Bushing Joint1/LConn1 -- Conn2/RConn1

== system robosimulador/Robô ==
  Lado Direito : Subsystem
  Lado Esquerdo : Subsystem
  Movimento : Subsystem
  Scope1 : Scope
  Scope3 : Scope
  Subsystem : Subsystem
  Subsystem1 : Subsystem
  Torso : Subsystem
  Conn1 : PMIOPort  Side=Left
  Chão : PMIOPort  Port=2  Side=Left
  CG : Outport  VectorParamsAs1DForOutWhenUnconnected=off
  ZMP : Outport  Port=2  VectorParamsAs1DForOutWhenUnconnected=off
  wires:
  Movimento/2(MOV PD) -> Lado Direito/1(Mov)
  Movimento/1(MOV PE) -> Lado Esquerdo/1(Mov)
  Subsystem/1(CG) -> CG/1, Scope3/1, Subsystem1/4(CGzmp)
  Subsystem1/1(ZMP) -> ZMP/1, Scope1/1
  Lado Direito/1(CG E) -> Subsystem/1(CG E)
  Lado Esquerdo/1(CG D) -> Subsystem/2(CG D)
  Torso/1(CG S) -> Subsystem/3(CG S)
  Torso/2(ZMP S) -> Subsystem1/3(ZMP S)
  Lado Direito/2(ZMP E) -> Subsystem1/1(ZMP E)
  Lado Esquerdo/2(ZMP D) -> Subsystem1/2(ZMP D)
  connections:
  Torso/LConn1 -- Conn1/RConn1
  Lado Esquerdo/LConn1 -- Torso/RConn1
  Lado Esquerdo/LConn2 -- Torso/RConn2
  Lado Direito/LConn1 -- Torso/RConn3
  Lado Direito/LConn2 -- Torso/RConn4
  Lado Esquerdo/LConn3 -- Lado Direito/LConn3 -- Chão/RConn1

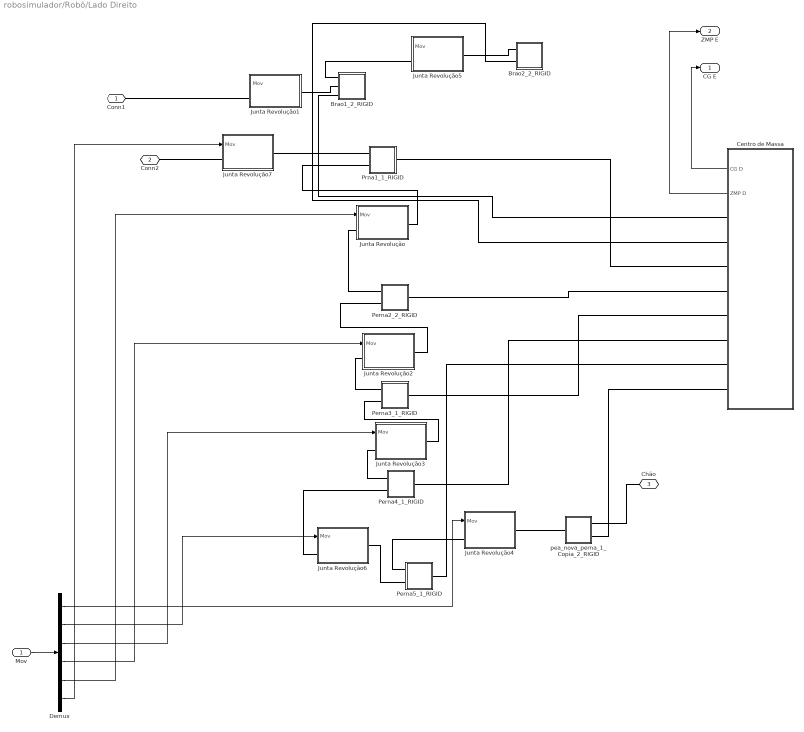
== system robosimulador/Robô/Lado Direito ==
  Mov : Inport
  Brao1_2_RIGID : Subsystem
  Brao2_2_RIGID : Subsystem
  Centro de Massa : Subsystem
  Demux : Demux  Outputs=6
  Junta Revolução : Subsystem
  Junta Revolução1 : Subsystem
  Junta Revolução2 : Subsystem
  Junta Revolução3 : Subsystem
  Junta Revolução4 : Subsystem
  Junta Revolução5 : Subsystem
  Junta Revolução6 : Subsystem
  Junta Revolução7 : Subsystem
  Perna2_2_RIGID : Subsystem
  Perna3_1_RIGID : Subsystem
  Perna4_1_RIGID : Subsystem
  Perna5_1_RIGID : Subsystem
  Prna1_1_RIGID : Subsystem
  pea_nova_perna_1_Copia_2_RIGID : Subsystem
  Conn1 : PMIOPort  Side=Left
  Conn2 : PMIOPort  Port=2  Side=Left
  Chão : PMIOPort  Port=3  Side=Left
  CG E : Outport  VectorParamsAs1DForOutWhenUnconnected=off
  ZMP E : Outport  Port=2  VectorParamsAs1DForOutWhenUnconnected=off
  wires:
  Mov/1 -> Demux/1
  Demux/1 -> Junta Revolução4/1(Mov)
  Demux/2 -> Junta Revolução6/1(Mov)
  Demux/3 -> Junta Revolução3/1(Mov)
  Demux/4 -> Junta Revolução2/1(Mov)
  Demux/5 -> Junta Revolução/1(Mov)
  Demux/6 -> Junta Revolução7/1(Mov)
  Centro de Massa/2(ZMP D) -> ZMP E/1
  Centro de Massa/1(CG D) -> CG E/1
  connections:
  Brao1_2_RIGID/LConn2 -- Junta Revolução1/RConn1
  Junta Revolução1/LConn1 -- Conn1/RConn1
  Perna2_2_RIGID/LConn1 -- Junta Revolução/LConn1
  Prna1_1_RIGID/LConn2 -- Junta Revolução/RConn1
  Perna3_1_RIGID/LConn1 -- Junta Revolução2/LConn1
  Junta Revolução2/RConn1 -- Perna2_2_RIGID/LConn2
  Perna4_1_RIGID/LConn1 -- Junta Revolução3/LConn1
  Perna3_1_RIGID/LConn2 -- Junta Revolução3/RConn1
  Perna5_1_RIGID/LConn1 -- Junta Revolução4/LConn1
  Junta Revolução4/RConn1 -- pea_nova_perna_1_Copia_2_RIGID/LConn1
  Brao1_2_RIGID/LConn1 -- Junta Revolução5/LConn1
  Brao2_2_RIGID/LConn1 -- Junta Revolução5/RConn1
  Perna5_1_RIGID/LConn2 -- Junta Revolução6/RConn1
  Junta Revolução6/LConn1 -- Perna4_1_RIGID/LConn2
  Prna1_1_RIGID/LConn1 -- Junta Revolução7/RConn1
  Junta Revolução7/LConn1 -- Conn2/RConn1
  Chão/RConn1 -- pea_nova_perna_1_Copia_2_RIGID/RConn1
  Brao1_2_RIGID/LConn3 -- Centro de Massa/RConn1
  Brao2_2_RIGID/LConn2 -- Centro de Massa/RConn2
  Prna1_1_RIGID/RConn1 -- Centro de Massa/RConn3
  Perna2_2_RIGID/RConn1 -- Centro de Massa/RConn4
  Perna3_1_RIGID/RConn1 -- Centro de Massa/RConn5
  Perna4_1_RIGID/RConn1 -- Centro de Massa/RConn6
  Perna5_1_RIGID/RConn1 -- Centro de Massa/RConn7
  pea_nova_perna_1_Copia_2_RIGID/RConn2 -- Centro de Massa/RConn8

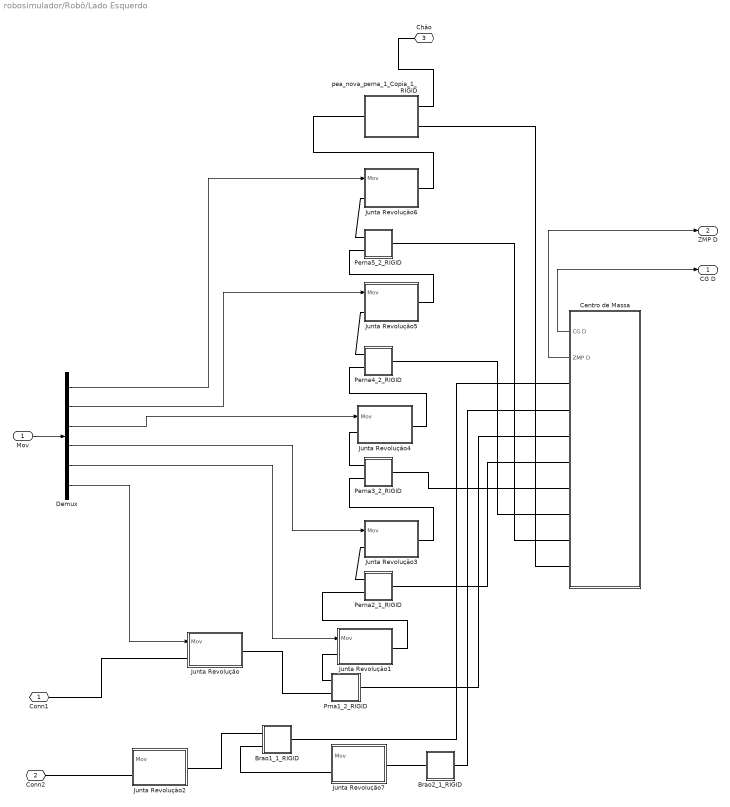
== system robosimulador/Robô/Lado Esquerdo ==
  Mov : Inport
  Brao1_1_RIGID : Subsystem
  Brao2_1_RIGID : Subsystem
  Centro de Massa : Subsystem
  Demux : Demux  Outputs=6
  Junta Revolução : Subsystem
  Junta Revolução1 : Subsystem
  Junta Revolução2 : Subsystem
  Junta Revolução3 : Subsystem
  Junta Revolução4 : Subsystem
  Junta Revolução5 : Subsystem
  Junta Revolução6 : Subsystem
  Junta Revolução7 : Subsystem
  Perna2_1_RIGID : Subsystem
  Perna3_2_RIGID : Subsystem
  Perna4_2_RIGID : Subsystem
  Perna5_2_RIGID : Subsystem
  Prna1_2_RIGID : Subsystem
  pea_nova_perna_1_Copia_1_RIGID : Subsystem
  Conn1 : PMIOPort  Side=Left
  Conn2 : PMIOPort  Port=2  Side=Left
  Chão : PMIOPort  Port=3  Side=Left
  CG D : Outport  VectorParamsAs1DForOutWhenUnconnected=off
  ZMP D : Outport  Port=2  VectorParamsAs1DForOutWhenUnconnected=off
  wires:
  Mov/1 -> Demux/1
  Demux/1 -> Junta Revolução6/1(Mov)
  Demux/2 -> Junta Revolução5/1(Mov)
  Demux/3 -> Junta Revolução4/1(Mov)
  Demux/4 -> Junta Revolução3/1(Mov)
  Demux/5 -> Junta Revolução1/1(Mov)
  Demux/6 -> Junta Revolução/1(Mov)
  Centro de Massa/2(ZMP D) -> ZMP D/1
  Centro de Massa/1(CG D) -> CG D/1
  connections:
  Perna2_1_RIGID/LConn2 -- Junta Revolução1/RConn1
  Brao1_1_RIGID/LConn1 -- Junta Revolução2/RConn1
  Junta Revolução/LConn1 -- Conn1/RConn1
  Junta Revolução2/LConn1 -- Conn2/RConn1
  Junta Revolução/RConn1 -- Prna1_2_RIGID/LConn2
  Prna1_2_RIGID/LConn1 -- Junta Revolução1/LConn1
  Perna2_1_RIGID/LConn1 -- Junta Revolução3/LConn1
  Junta Revolução3/RConn1 -- Perna3_2_RIGID/LConn2
  Perna3_2_RIGID/LConn1 -- Junta Revolução4/LConn1
  Junta Revolução4/RConn1 -- Perna4_2_RIGID/LConn2
  Perna4_2_RIGID/LConn1 -- Junta Revolução5/LConn1
  Junta Revolução5/RConn1 -- Perna5_2_RIGID/LConn2
  Perna5_2_RIGID/LConn1 -- Junta Revolução6/LConn1
  Junta Revolução6/RConn1 -- pea_nova_perna_1_Copia_1_RIGID/LConn1
  Brao1_1_RIGID/LConn2 -- Junta Revolução7/LConn1
  Junta Revolução7/RConn1 -- Brao2_1_RIGID/LConn1
  pea_nova_perna_1_Copia_1_RIGID/RConn1 -- Chão/RConn1
  Brao1_1_RIGID/RConn1 -- Centro de Massa/RConn1
  Brao2_1_RIGID/RConn1 -- Centro de Massa/RConn2
  Prna1_2_RIGID/RConn1 -- Centro de Massa/RConn3
  Perna2_1_RIGID/RConn1 -- Centro de Massa/RConn4
  Perna3_2_RIGID/RConn1 -- Centro de Massa/RConn5
  Perna4_2_RIGID/RConn1 -- Centro de Massa/RConn6
  Perna5_2_RIGID/RConn1 -- Centro de Massa/RConn7
  pea_nova_perna_1_Copia_1_RIGID/RConn2 -- Centro de Massa/RConn8

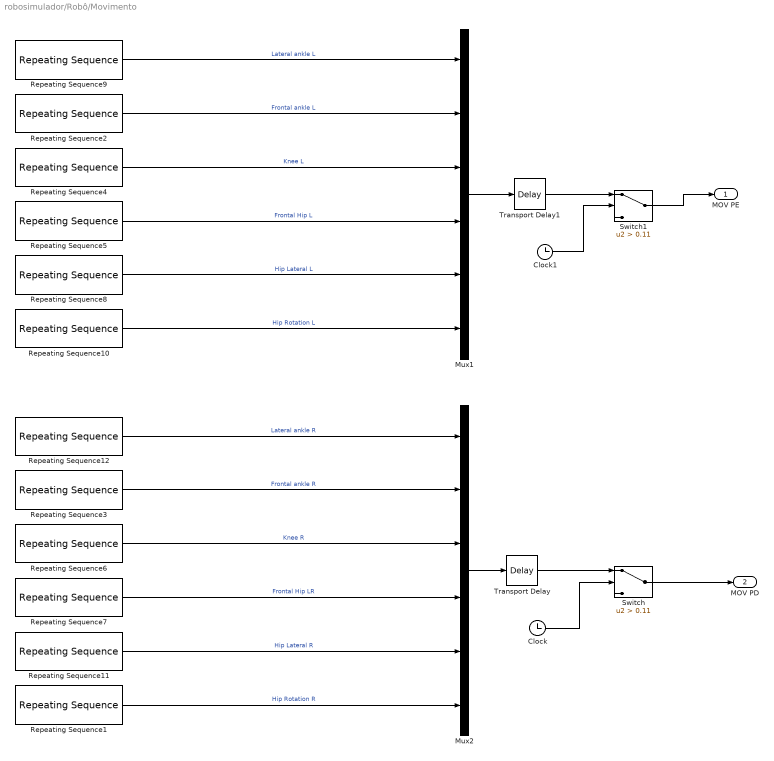
== system robosimulador/Robô/Movimento ==
  Clock : Clock
  Clock1 : Clock
  Mux1 : Mux  Inputs=6
  Mux2 : Mux  Inputs=6
  Repeating Sequence1 : simulink/Sources/Repeating Sequence  rep_seq_t=Time(1:j)  rep_seq_y=Q(1:j,6)
  Repeating Sequence10 : simulink/Sources/Repeating Sequence  rep_seq_t=Time(1:j)  rep_seq_y=Q(1:j,7)
  Repeating Sequence11 : simulink/Sources/Repeating Sequence  rep_seq_t=Time(1:j)  rep_seq_y=Q(1:j,5)
  Repeating Sequence12 : simulink/Sources/Repeating Sequence  rep_seq_t=Time(1:j)  rep_seq_y=Q(1:j,1)
  Repeating Sequence2 : simulink/Sources/Repeating Sequence  rep_seq_t=Time(1:j)  rep_seq_y=Q(1:j,11)
  Repeating Sequence3 : simulink/Sources/Repeating Sequence  rep_seq_t=Time(1:j)  rep_seq_y=Q(1:j,2)
  Repeating Sequence4 : simulink/Sources/Repeating Sequence  rep_seq_t=Time(1:j)  rep_seq_y=Q(1:j,10)
  Repeating Sequence5 : simulink/Sources/Repeating Sequence  rep_seq_t=Time(1:j)  rep_seq_y=Q(1:j,9)
  Repeating Sequence6 : simulink/Sources/Repeating Sequence  rep_seq_t=Time(1:j)  rep_seq_y=Q(1:j,3)
  Repeating Sequence7 : simulink/Sources/Repeating Sequence  rep_seq_t=Time(1:j)  rep_seq_y=Q(1:j,4)
  Repeating Sequence8 : simulink/Sources/Repeating Sequence  rep_seq_t=Time(1:j)  rep_seq_y=Q(1:j,8)
  Repeating Sequence9 : simulink/Sources/Repeating Sequence  rep_seq_t=Time(1:j)  rep_seq_y=Q(1:j,12)
  Switch : Switch  Criteria=u2 > Threshold  Threshold=0.11
  Switch1 : Switch  Criteria=u2 > Threshold  Threshold=0.11
  Transport Delay : TransportDelay  DelayTime=0.11
  Transport Delay1 : TransportDelay  DelayTime=0.11
  MOV PE : Outport  VectorParamsAs1DForOutWhenUnconnected=off
  MOV PD : Outport  Port=2  VectorParamsAs1DForOutWhenUnconnected=off
  wires:
  Clock/1 -> Switch/2
  Switch/1 -> MOV PD/1
  Switch1/1 -> MOV PE/1
  Clock1/1 -> Switch1/2
  Transport Delay/1 -> Switch/1
  Mux1/1 -> Transport Delay1/1
  Transport Delay1/1 -> Switch1/1
  Repeating Sequence9/1 -> Mux1/1  "Lateral ankle L"
  Repeating Sequence2/1 -> Mux1/2  "Frontal ankle L"
  Repeating Sequence4/1 -> Mux1/3  "Knee L"
  Repeating Sequence5/1 -> Mux1/4  "Frontal Hip L"
  Repeating Sequence8/1 -> Mux1/5  "Hip Lateral L"
  Repeating Sequence10/1 -> Mux1/6  "Hip Rotation L"
  Repeating Sequence12/1 -> Mux2/1  "Lateral ankle R"
  Repeating Sequence6/1 -> Mux2/3  "Knee R"
  Repeating Sequence11/1 -> Mux2/5  "Hip Lateral R"
  Repeating Sequence1/1 -> Mux2/6  "Hip Rotation R"
  Repeating Sequence3/1 -> Mux2/2  "Frontal ankle R"
  Repeating Sequence7/1 -> Mux2/4  "Frontal Hip LR"
  Mux2/1 -> Transport Delay/1

== system robosimulador/Robô/Subsystem ==
  CG E : Inport
  CG D : Inport  Port=2
  CG S : Inport  Port=3
  Centro de massa : Subsystem
  CG : Outport  VectorParamsAs1DForOutWhenUnconnected=off
  wires:
  Centro de massa/1("CM ") -> CG/1
  CG D/1 -> Centro de massa/1(CG D)
  CG S/1 -> Centro de massa/3(CG S)
  CG E/1 -> Centro de massa/2(CG E)

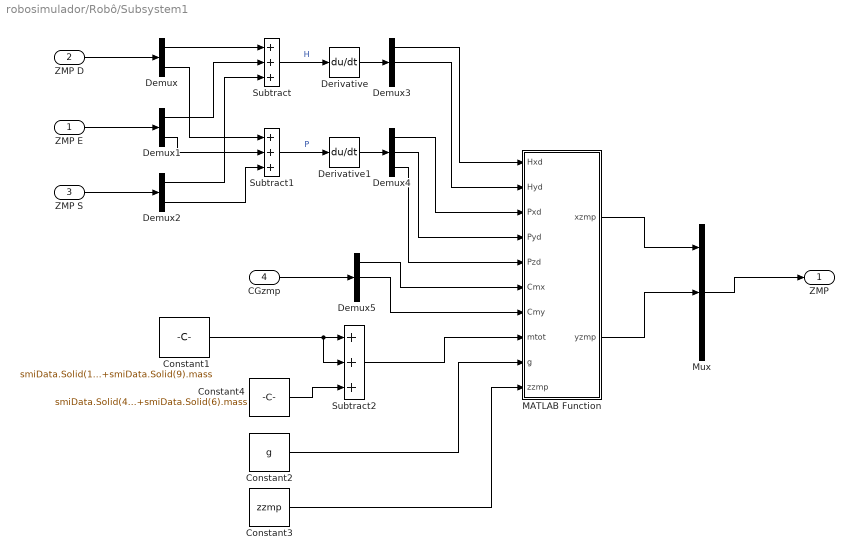
== system robosimulador/Robô/Subsystem1 ==
  ZMP E : Inport
  ZMP D : Inport  Port=2
  ZMP S : Inport  Port=3
  CGzmp : Inport  Port=4
  Constant1 : Constant  Value=smiData.Solid(1).mass+smiData.Solid(2).mass+smiData.Solid(3).mass+smiData.Solid(10).mass+smiData.Solid(5).mass+smiData.Solid(7).mass+smiData.Solid(11).mass+smiData.Solid(9).mass
  Constant2 : Constant  Value=g
  Constant3 : Constant  Value=zzmp
  Constant4 : Constant  Value=smiData.Solid(4).mass+smiData.Solid(6).mass
  Demux : Demux  Outputs=2
  Demux1 : Demux  Outputs=2
  Demux2 : Demux  Outputs=2
  Demux3 : Demux  Outputs=3
  Demux4 : Demux  Outputs=3
  Demux5 : Demux  Outputs=3
  Derivative : Derivative
  Derivative1 : Derivative
  MATLAB Function : MATLAB Function  TreatAsAtomicUnit=on
  Mux : Mux  Inputs=3
  Subtract : Sum  Inputs=+++
  Subtract1 : Sum  Inputs=+++
  Subtract2 : Sum  Inputs=+++
  ZMP : Outport  VectorParamsAs1DForOutWhenUnconnected=off
  wires:
  ZMP E/1 -> Demux1/1
  ZMP S/1 -> Demux2/1
  ZMP D/1 -> Demux/1
  Demux/1 -> Subtract/1
  Demux1/1 -> Subtract/2
  Demux2/1 -> Subtract/3
  Demux/2 -> Subtract1/1
  Demux1/2 -> Subtract1/2
  Demux2/2 -> Subtract1/3
  Subtract/1 -> Derivative/1  "H"
  Subtract1/1 -> Derivative1/1  "P"
  CGzmp/1 -> Demux5/1
  Constant1/1 -> Subtract2/2, Subtract2/1
  Constant4/1 -> Subtract2/3
  Derivative/1 -> Demux3/1
  Derivative1/1 -> Demux4/1
  Demux3/1 -> MATLAB Function/1(Hxd)
  Demux3/2 -> MATLAB Function/2(Hyd)
  Demux4/1 -> MATLAB Function/3(Pxd)
  Demux4/2 -> MATLAB Function/4(Pyd)
  Demux4/3 -> MATLAB Function/5(Pzd)
  Demux5/1 -> MATLAB Function/6(Cmx)
  Demux5/2 -> MATLAB Function/7(Cmy)
  Subtract2/1 -> MATLAB Function/8(mtot)
  Constant2/1 -> MATLAB Function/9(g)
  Constant3/1 -> MATLAB Function/10(zzmp)
  MATLAB Function/1(xzmp) -> Mux/1
  MATLAB Function/2(yzmp) -> Mux/2
  Mux/1 -> ZMP/1

== system robosimulador/Robô/Torso ==
  Cabea1_1_RIGID : Subsystem
  Cabea2_1_RIGID : Subsystem
  CoM e ZMP Superior : Subsystem
  Torso1_1_RIGID : Subsystem
  Conn1 : PMIOPort  Side=Left
  Conn2 : PMIOPort  Port=2  Side=Right
  Connn3 : PMIOPort  Port=3  Side=Right
  Conn : PMIOPort  Port=4  Side=Right
  Conn5 : PMIOPort  Port=5  Side=Right
  CG S : Outport
  ZMP S : Outport  Port=2
  wires:
  CoM e ZMP Superior/1(CG S) -> CG S/1
  CoM e ZMP Superior/2(ZMP S) -> ZMP S/1
  connections:
  Conn/RConn1 -- Torso1_1_RIGID/LConn2
  Conn2/RConn1 -- Torso1_1_RIGID/LConn1
  Connn3/RConn1 -- Torso1_1_RIGID/LConn3
  Conn5/RConn1 -- Torso1_1_RIGID/LConn4
  Cabea1_1_RIGID/LConn1 -- Conn1/RConn1
  Cabea1_1_RIGID/LConn2 -- Cabea2_1_RIGID/LConn1
  Cabea2_1_RIGID/LConn2 -- Torso1_1_RIGID/RConn1
  Torso1_1_RIGID/RConn2 -- CoM e ZMP Superior/RConn1
  Cabea1_1_RIGID/RConn1 -- CoM e ZMP Superior/RConn2
  Cabea2_1_RIGID/RConn1 -- CoM e ZMP Superior/RConn3
